simulink model "Retro_de_estados_RMS"  (R2020a)
settings: Solver=VariableStepAuto  StartTime=0.0  StopTime=10.0  MaxStep=0.0001  RelTol=1e-3
undefined symbols (not defined in the file): Amp, bm, K, K_motor, k_resorte, Ki, kr, L, m_total, R
libraries: dspstat3 x1
settings Model: Creator=Adriana  LastModifiedBy=Noxi-PC

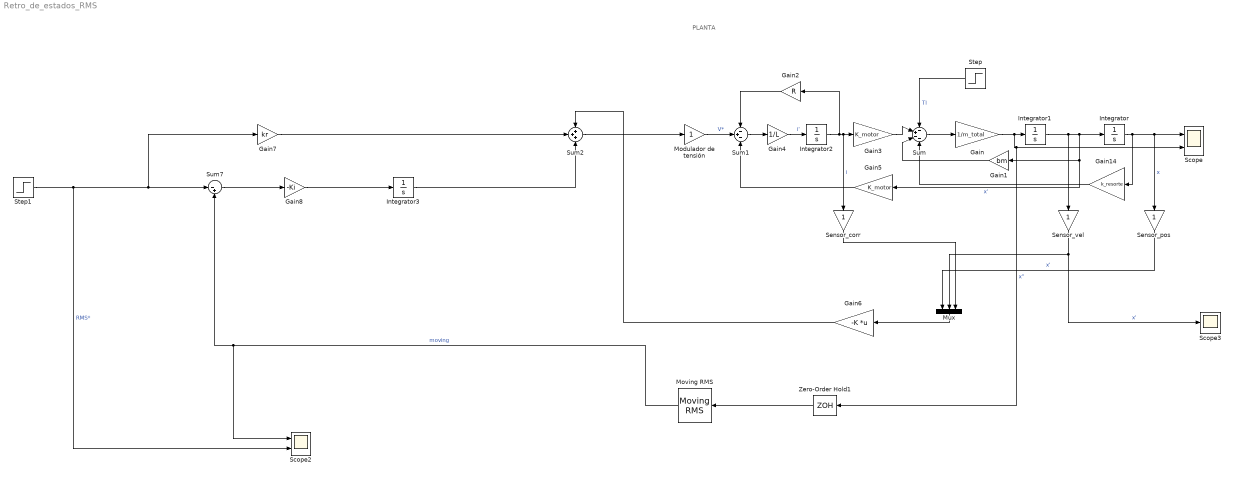
== system Retro_de_estados_RMS ==
  note: PLANTA
  " Sensor_pos" : Gain
  " Sensor_vel" : Gain
  Gain : Gain  Gain=1/m_total
  Gain1 : Gain  Gain=bm
  Gain14 : Gain  Gain=k_resorte
  Gain2 : Gain  Gain=R
  Gain3 : Gain  Gain=K_motor
  Gain4 : Gain  Gain=1/L
  Gain5 : Gain  Gain=K_motor
  Gain6 : Gain  Gain=-K  Multiplication=Matrix(K*u)
  Gain7 : Gain  Gain=kr
  Gain8 : Gain  Gain=-Ki
  Integrator{,1..3} (4 alike) : Integrator
  Modulador de tensión : Gain
  Moving RMS : dspstat3/Moving RMS  Method=Sliding window  ForgettingFactorPort=off  SpecifyWindowLength=on  WindowLength=Ventana  ForgettingFactor=0.99  SimulateUsing=Code generation
      settings: SourceProductBaseCode=DS
  Mux : Mux  Inputs=3
  Scope : Scope  NumInputPorts=2
  Scope2 : Scope  NumInputPorts=2
  Scope3 : Scope
  Sensor_corr : Gain
  Step : Step  Time=3  After=0  SampleTime=0
  Step1 : Step  After=Amp/sqrt(2)  SampleTime=0
  Sum : Sum  Inputs=-+--
  Sum1 : Sum  Inputs=-+-
  Sum2 : Sum  Inputs=+++
  Sum7 : Sum  Inputs=|-+
  Zero-Order Hold1 : ZeroOrderHold  SampleTime=-1
  wires:
  Integrator1/1 -> " Sensor_vel"/1, Gain5/1, Gain1/1, Integrator/1  "x'"
  Integrator/1 -> Gain14/1, " Sensor_pos"/1, Scope/1  "x"
  Gain/1 -> Scope/2, Zero-Order Hold1/1, Integrator1/1  "x''"
  Sum/1 -> Gain/1
  Gain1/1 -> Sum/3
  Step/1 -> Sum/1  "Tl"
  Gain3/1 -> Sum/2
  Integrator2/1 -> Gain2/1, Gain3/1, Sensor_corr/1  "i"
  Sum1/1 -> Gain4/1
  Gain4/1 -> Integrator2/1  "i'"
  Gain2/1 -> Sum1/1
  Gain5/1 -> Sum1/3
  Modulador de tensión/1 -> Sum1/2  "V*"
  " Sensor_vel"/1 -> Mux/2, Scope3/1  "x'"
  Gain14/1 -> Sum/4
  Moving RMS/1 -> Scope2/1, Sum7/2  "moving"
  Zero-Order Hold1/1 -> Moving RMS/1
  Step1/1 -> Scope2/2, Gain7/1, Sum7/1  "RMS*"
  " Sensor_pos"/1 -> Mux/1  "x'"
  Sensor_corr/1 -> Mux/3
  Mux/1 -> Gain6/1
  Sum2/1 -> Modulador de tensión/1
  Gain7/1 -> Sum2/2
  Gain6/1 -> Sum2/1
  Sum7/1 -> Gain8/1
  Gain8/1 -> Integrator3/1
  Integrator3/1 -> Sum2/3
